simulink model "WS4_SIMmodel_v2017b"  (R2019b)
settings: Solver=VariableStepAuto  StartTime=0.0  StopTime=15  MaxStep=0.05  RelTol=1e-6
values from neighbouring files (symbols this model uses):
  initcond = [0; -0.05; 0; 0]    [WS4_SIMmodel_param.m]
  K = 1    [WS4_SIMmodel_param.m]
  pendCden = [0.0095564 1]    [WS4_SIMmodel_param.m]
  pendCnum = 5276.04 * [0.1163 1]    [WS4_SIMmodel_param.m]
  SqWaveFreq = 1/18    (= 0.0555555555556)    [WS4_SIMmodel_param.m]
  ThDotRef = 90    [WS4_SIMmodel_param.m]
  ThRef = 45    [WS4_SIMmodel_param.m]
undefined symbols (not defined in the file or in its folder): qdotmobpend
settings Model: Creator=mwcant  LastModifiedBy=linesLK
settings DebuggingCC: ArithmeticOperatorsInVariantConditions=warning
settings SFSimCC: CustomCodeUndefinedFunction=UseInterfaceOnly

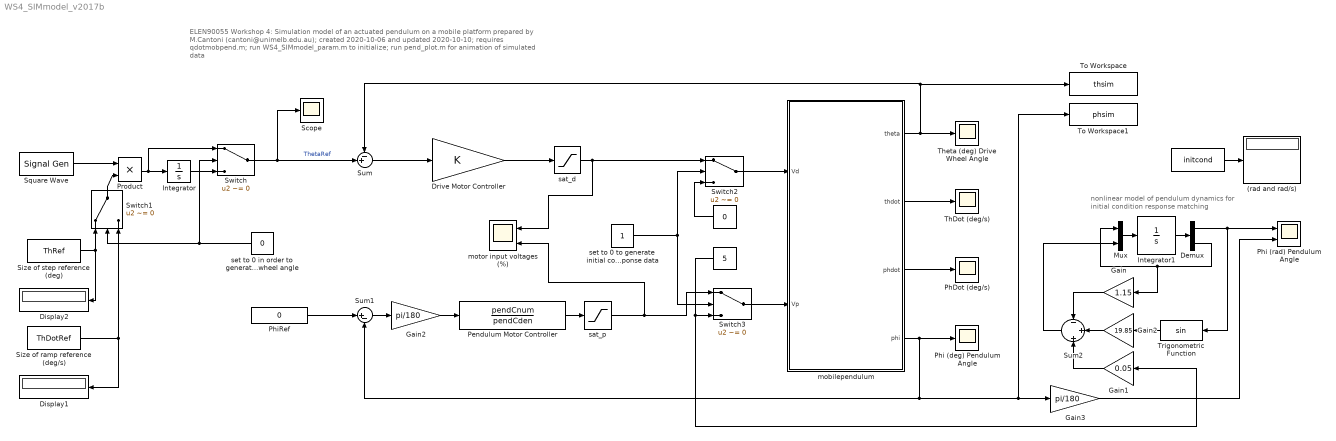
== system WS4_SIMmodel_v2017b ==
  note: ELEN90055 Workshop 4: Simulation model of an actuated pendulum on a mobile platform
      | prepared by M.Cantoni (cantoni@unimelb.edu.au); created 2020-10-06 and updated 2020-10-10; requires qdotmobpend.m; run WS4_SIMmodel_param.m to initialize; run pend_plot.m for animation of simulated data
  note: nonlinear model of pendulum dynamics
      | for initial condition response matching
  " " : Constant  Value=0
  "   " : Constant  Value=5
  "    " : Constant  Value=initcond
  (rad and rad/s) : Display
  Demux : Demux  Outputs=2
  Display1 : Display
  Display2 : Display
  Drive Motor Controller : Gain  Gain=K
  Gain : Gain  Gain=1.15
  Gain1 : Gain  Gain=0.05
  Gain2 : Gain  Gain=pi/180
  "Gain2 " : Gain  Gain=19.85
  Gain3 : Gain  Gain=pi/180
  Integrator : Integrator
  Integrator1 : Integrator  InitialCondition=[initcond(2);initcond(4)]
  Mux : Mux  Inputs=2
  Pendulum Motor Controller : TransferFcn  Numerator=pendCnum  Denominator=pendCden
  PhDot (deg/s) : Scope
  Phi (deg) Pendulum Angle : Scope
  Phi (rad) Pendulum Angle : Scope  NumInputPorts=2
  PhiRef : Constant  Value=0
  Product : Product
  Scope : Scope
  Size of ramp reference (deg/s) : Constant  Value=ThDotRef
  Size of step reference (deg) : Constant  Value=ThRef
  Square Wave : SignalGenerator  WaveForm=square  Frequency=SqWaveFreq
  Sum : Sum  Inputs=-+|
  Sum1 : Sum  Inputs=|+-
  Sum2 : Sum  Inputs=-|+|+
  Switch{,1..3} (4 alike) : Switch  Criteria=u2 ~= 0
  ThDot (deg/s) : Scope
  Theta (deg) Drive Wheel Angle : Scope
  To Workspace : ToWorkspace  VariableName=thsim  SaveFormat=Timeseries  SampleTime=-1
  To Workspace1 : ToWorkspace  VariableName=phsim  SaveFormat=Timeseries  SampleTime=-1
  Trigonometric Function : Trigonometry
  "mobilependulum " : Subsystem
  "motor input voltages (%) " : Scope  NumInputPorts=2
  sat_d : Saturate  UpperLimit=100  LowerLimit=-100
  "sat_p " : Saturate  UpperLimit=100  LowerLimit=-100
  set to 0 in order to generate triangle (instead of square)  wave reference for the drive wheel angle : Constant  Value=0
  set to 0 to generate initial condition response data : Constant
  wires:
  PhiRef/1 -> Sum1/1
  "mobilependulum "/3(phdot) -> PhDot (deg/s)/1
  Sum/1 -> Drive Motor Controller/1
  Sum1/1 -> Gain2/1
  "mobilependulum "/1(theta) -> Theta (deg) Drive Wheel Angle/1, To Workspace/1, Sum/1
  Product/1 -> Switch/1, Integrator/1
  "mobilependulum "/2(thdot) -> ThDot (deg/s)/1
  Square Wave/1 -> Product/1
  sat_d/1 -> Switch2/1, "motor input voltages (%) "/1
  "mobilependulum "/4(phi) -> Phi (deg) Pendulum Angle/1, To Workspace1/1, Gain3/1, Sum1/2
  Pendulum Motor Controller/1 -> "sat_p "/1
  Drive Motor Controller/1 -> sat_d/1
  Switch/1 -> Scope/1, Sum/2  "ThetaRef"
  Integrator/1 -> Switch/3
  Switch1/1 -> Product/2
  Size of ramp reference (deg/s)/1 -> Switch1/3, Display1/1
  Size of step reference (deg)/1 -> Switch1/1, Display2/1
  set to 0 in order to generate triangle (instead of square)  wave reference for the drive wheel angle/1 -> Switch1/2, Switch/2
  Switch2/1 -> "mobilependulum "/1(Vd)
  Switch3/1 -> "mobilependulum "/2(Vp)
  set to 0 to generate initial condition response data/1 -> Switch2/2, Switch3/2
  "sat_p "/1 -> Switch3/1, "motor input voltages (%) "/2
  Integrator1/1 -> Demux/1
  Mux/1 -> Integrator1/1
  Trigonometric Function/1 -> "Gain2 "/1
  Demux/2 -> Mux/1, Gain/1
  Sum2/1 -> Mux/2
  Gain/1 -> Sum2/1
  Demux/1 -> Trigonometric Function/1, Phi (rad) Pendulum Angle/1
  " "/1 -> Switch2/3
  Gain3/1 -> Phi (rad) Pendulum Angle/2
  "   "/1 -> Switch3/3, Gain1/1
  "    "/1 -> (rad and rad/s)/1
  "Gain2 "/1 -> Sum2/2
  Gain1/1 -> Sum2/3
  Gain2/1 -> Pendulum Motor Controller/1

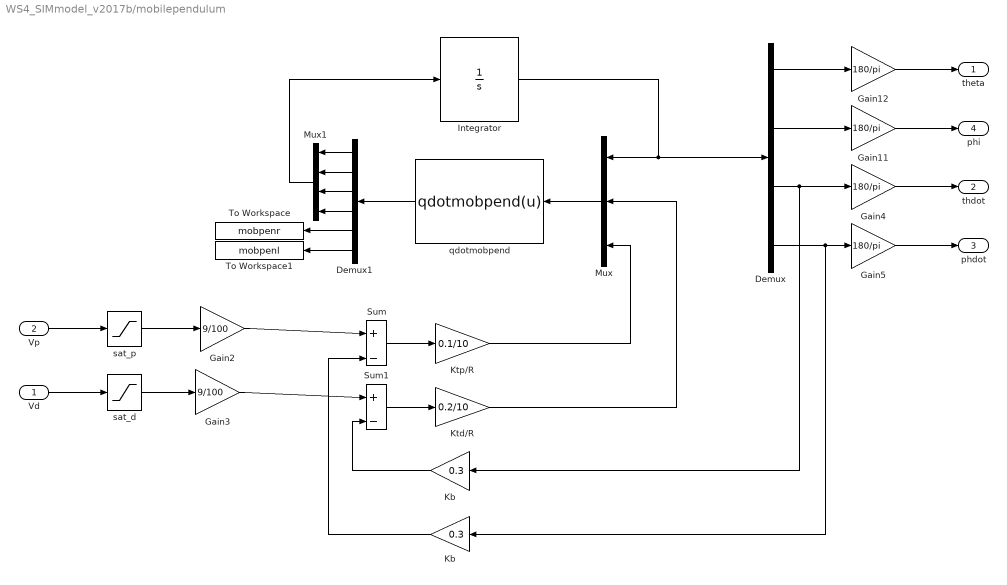
== system WS4_SIMmodel_v2017b/mobilependulum  ==
  Vd : Inport
  Vp : Inport  Port=2
  Demux : Demux
  Demux1 : Demux  Outputs=6
  Gain{4..5,11..12} (4 alike) : Gain  Gain=180/pi
  Gain2 : Gain  Gain=9/100
  Gain3 : Gain  Gain=9/100
  Integrator : Integrator  InitialCondition=initcond
  Kb : Gain  Gain=0.3
  "Kb " : Gain  Gain=0.3
  "Ktd/R " : Gain  Gain=0.2/10
  Ktp/R : Gain  Gain=0.1/10
  Mux : Mux  Inputs=3
  Mux1 : Mux
  Sum : Sum  Inputs=+|-
  Sum1 : Sum  Inputs=+|-
  To Workspace : ToWorkspace  VariableName=mobpenr  SampleTime=-1
      settings: Save2DSignal=2-D array (concatenate along first dimension)
  To Workspace1 : ToWorkspace  VariableName=mobpenl  SampleTime=-1
      settings: Save2DSignal=2-D array (concatenate along first dimension)
  qdotmobpend : MATLABFcn  MATLABFcn=qdotmobpend(u)
  sat_d : Saturate  UpperLimit=100  LowerLimit=-100
  "sat_p " : Saturate  UpperLimit=100  LowerLimit=-100
  theta : Outport
  thdot : Outport  Port=2
  phdot : Outport  Port=3
  phi : Outport  Port=4
  wires:
  Vp/1 -> "sat_p "/1
  Vd/1 -> sat_d/1
  Demux/1 -> Gain12/1
  Sum/1 -> Ktp/R/1
  Mux/1 -> qdotmobpend/1
  Integrator/1 -> Mux/1, Demux/1
  Sum1/1 -> "Ktd/R "/1
  Demux/2 -> Gain11/1
  Kb/1 -> Sum1/2
  "sat_p "/1 -> Gain2/1
  sat_d/1 -> Gain3/1
  Gain3/1 -> Sum1/1
  Demux/3 -> Kb/1, Gain4/1
  Gain4/1 -> thdot/1
  Gain5/1 -> phdot/1
  Demux/4 -> "Kb "/1, Gain5/1
  Gain11/1 -> phi/1
  Gain12/1 -> theta/1
  "Ktd/R "/1 -> Mux/2
  "Kb "/1 -> Sum/2
  Ktp/R/1 -> Mux/3
  Gain2/1 -> Sum/1
  qdotmobpend/1 -> Demux1/1
  Demux1/1 -> Mux1/1
  Demux1/2 -> Mux1/2
  Demux1/3 -> Mux1/3
  Demux1/4 -> Mux1/4
  Mux1/1 -> Integrator/1
  Demux1/5 -> To Workspace/1
  Demux1/6 -> To Workspace1/1
